simulink model "heart_model"  (Simulink 8.5)
settings: Solver=ode3  StartTime=0.0  StopTime=size(sasignal,1)  FixedStep=1  RelTol=1e-6  AbsTol=1e-6
undefined symbols (not defined in the file or in its folder): beta1, beta3, beta4, delay, gain
libraries: simulink x40, dspsrcs4 x1
(part 1 of 5)
CloseFcn:
  | rtwprivate ssgensfun ModelCloseRequest cellblocksimfast
settings Model: Creator=mereacre  LastModifiedBy=piergiuseppe  CovSFcnEnable=off
settings DataIOCC: LimitDataPoints=off  SaveOutput=off  SignalLogging=off  DSMLogging=off  SaveTime=off
settings DebuggingCC: SolverPrmCheckMsg=warning  MultiTaskDSMMsg=warning  MultiTaskCondExecSysMsg=none  FcnCallInpInsideContextMsg=EnableAllAsError
settings RTWCC: RTWCompilerOptimization=on

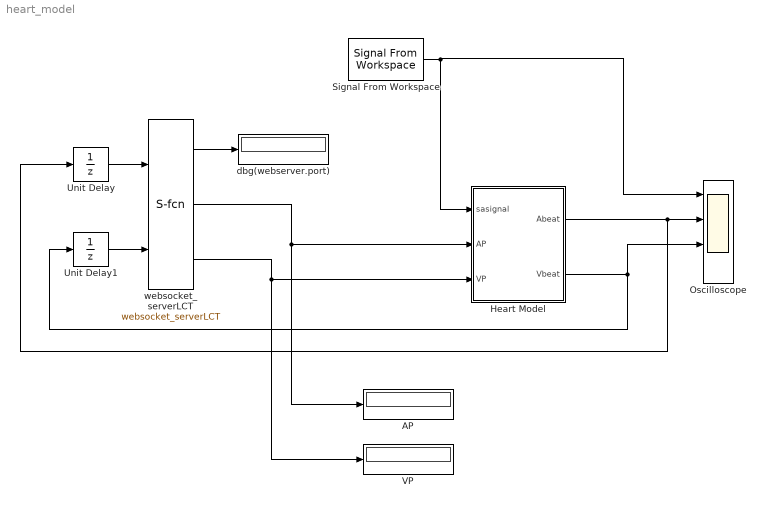
== system heart_model ==
  AP : Display
  Heart Model : Subsystem
  Oscilloscope : Scope  NumInputPorts=4
      settings: TimeRange=16384  YMin=-5~-5~-5~-5  YMax=2~5~5~5
  Signal From Workspace : dspsrcs4/Signal From Workspace  X=sasignal  Ts=1  nsamps=1  OutputAfterFinalValue=Setting to zero  ignoreOrWarnInputAndFrameLengths=off
  Unit Delay : UnitDelay  SampleTime=-1
  Unit Delay1 : UnitDelay  SampleTime=-1
  "VP " : Display
  dbg(webserver.port) : Display
  websocket_serverLCT : S-Function  FunctionName=websocket_serverLCT  mask(Legacy Function){SFunctionSpec=uint32 y1 = WebsocketServer(double u1, double u2, uint32 y2[1], uint32 y3[1]), ShowSpec=on}
      mask prompts: ShowSpec "Display function specification"
      mask help:
      | This block allows you to call the legacy functions specified by the following Legacy Code Tool definition:
      | def.SFunctionName = 'websocket_serverLCT';
      | def.OutputFcnSpec = 'uint32 y1 = WebsocketServer(double u1, double u2, uint32 y2[1], uint32 y3[1])';
      | def.TerminateFcnSpec = 'close_websocket()';
      | def.HeaderFiles = {'websocket_server.h'};
      | def.SourceFiles = {'websocket_server.c'};
      | def.HostLibFiles = {'libwebsockets.dylib'};
      mask Help: <p>This block was generated automatically by the Legacy Code Tool. For detailed help on this tool, call<a href="matlab:legacy_code('help')"> legacy_code('help')</a>.</p>
      mask Callback ShowSpec:
      | if strcmp(get_param(gcbh, 'ShowSpec'), 'on')
      |   set_param(gcbh, 'MaskDisplay', sprintf('fprintf(''%s'');', get_param(gcbh, 'SFunctionSpec')));
      | else
      |   set_param(gcbh, 'MaskDisplay', sprintf('fprintf(''%s'');', get_param(gcbh, 'FunctionName')));
      | end
      mask Display: fprintf('uint32 y1 = WebsocketServer(double u1, double u2, uint32 y2[1], uint32 y3[1])');
  wires:
  Signal From Workspace/1 -> Heart Model/1(sasignal), Oscilloscope/1
  Heart Model/2(Vbeat) -> Oscilloscope/3, Unit Delay1/1
  Heart Model/1(Abeat) -> Oscilloscope/2, Unit Delay/1
  Unit Delay1/1 -> websocket_serverLCT/2
  Unit Delay/1 -> websocket_serverLCT/1
  websocket_serverLCT/2 -> AP/1, Heart Model/2(AP)
  websocket_serverLCT/3 -> "VP "/1, Heart Model/3(VP)
  websocket_serverLCT/1 -> dbg(webserver.port)/1

== system heart_model/Heart Model ==
  sasignal : Inport
  AP : Inport  Port=2
  VP : Inport  Port=3
  ATRIUM : Subsystem
  AV (3) : Subsystem
  Action Threshold : Subsystem
  Action Threshold1 : Subsystem
  Action Threshold2 : Subsystem
  Channel ID : Constant  Value=2
  Channel ID1 : Constant  Value=2
  Constant26 : Constant  Value=0
  Constant27 : Constant  Value=gain(3)
  I_st : Constant  Value=0.7
  SA (1) : Subsystem
  VENTRICLE : Subsystem
  vin : Constant  Value=0
  Abeat : Outport
  Vbeat : Outport  Port=2
  wires:
  ATRIUM/2(scope_out) -> Action Threshold/1(v)
  Channel ID1/1 -> VENTRICLE/2(scope_in1)
  AV (3)/1(vout) -> VENTRICLE/1(vin)
  Constant27/1 -> AV (3)/4(win)
  ATRIUM/1(vout) -> AV (3)/3(vin)
  Constant26/1 -> AV (3)/2(I_st), AV (3)/1(stim)
  Channel ID/1 -> ATRIUM/2(scope_in)
  SA (1)/1(vout) -> ATRIUM/1(vin)
  vin/1 -> SA (1)/4(win), SA (1)/3(vin)
  I_st/1 -> SA (1)/2(I_st)
  sasignal/1 -> SA (1)/1(stim)
  Action Threshold/1(Aget) -> Abeat/1  "Agetsig"
  AP/1 -> ATRIUM/3(stim)
  VP/1 -> VENTRICLE/3(stim)
  VENTRICLE/1(scope_out) -> Action Threshold1/1(v), Action Threshold2/1(v)
  Action Threshold1/1(Aget) -> Vbeat/1

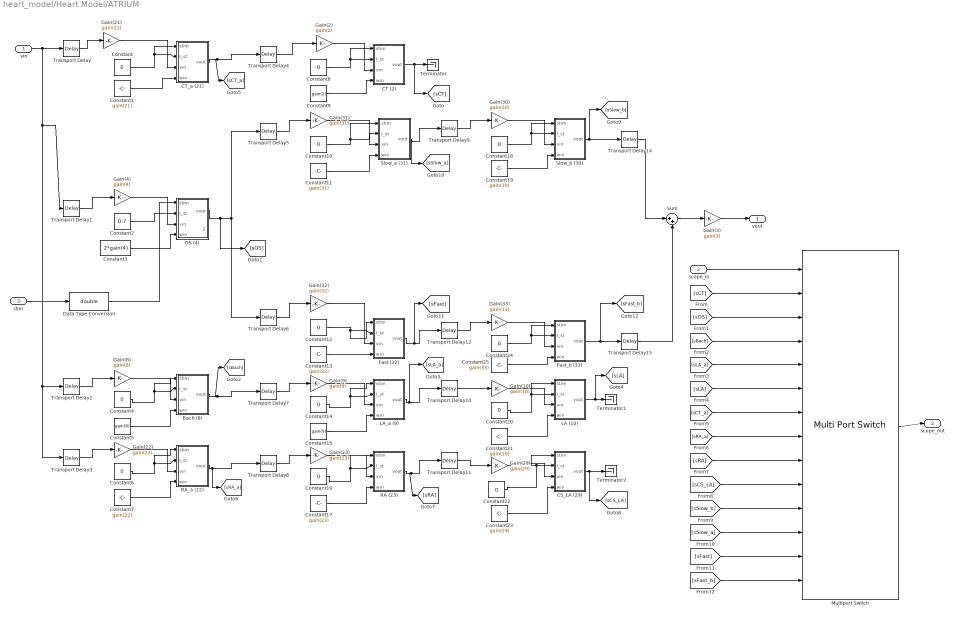
== system heart_model/Heart Model/ATRIUM ==
  vin : Inport
  scope_in : Inport  Port=2
  stim : Inport  Port=3
  Bach (8) : Subsystem
  CS_LA (29) : Subsystem
  CT (2) : Subsystem
  CT_a (21) : Subsystem
  Constant{,4,6,8,10,12,14,16,18,20,22,24} (12 alike) : Constant  Value=0
  Constant1 : Constant  Value=gain(21)
  Constant11 : Constant  Value=gain(31)
  Constant13 : Constant  Value=gain(32)
  Constant15 : Constant  Value=gain(9)
  Constant17 : Constant  Value=gain(23)
  Constant19 : Constant  Value=gain(30)
  Constant2 : Constant  Value=0.7
  Constant21 : Constant  Value=gain(10)
  Constant23 : Constant  Value=gain(29)
  Constant25 : Constant  Value=gain(33)
  Constant3 : Constant  Value=2*gain(4)
  Constant5 : Constant  Value=gain(8)
  Constant7 : Constant  Value=gain(22)
  Constant9 : Constant  Value=gain(2)
  Data Type Conversion : DataTypeConversion  OutMin=[0]  OutMax=[1]  OutDataTypeStr=double
  Fast (32) : Subsystem
  Fast_b (33) : Subsystem
  Gain(10) : Gain  Gain=gain(10)
  Gain(2) : Gain  Gain=gain(2)
  Gain(21) : Gain  Gain=gain(21)
  Gain(22) : Gain  Gain=gain(22)
  Gain(23) : Gain  Gain=gain(23)
  Gain(29) : Gain  Gain=gain(29)
  Gain(3) : Gain  Gain=gain(3)
  Gain(30) : Gain  Gain=gain(30)
  Gain(31) : Gain  Gain=gain(31)
  Gain(32) : Gain  Gain=gain(32)
  Gain(33) : Gain  Gain=gain(33)
  Gain(4) : Gain  Gain=gain(4)
  Gain(8) : Gain  Gain=gain(8)
  Gain(9) : Gain  Gain=gain(9)
  LA (10) : Subsystem
  LA_a (9) : Subsystem
  Multiport Switch : MultiPortSwitch  Inputs=13
  OS (4) : Subsystem
  RA (23) : Subsystem
  RA_a (22) : Subsystem
  Slow_a (31) : Subsystem
  Slow_b (30) : Subsystem
  Sum : Sum  Inputs=|++
  Terminator : Terminator
  Terminator1 : Terminator
  Terminator2 : Terminator
  Transport Delay : TransportDelay  DelayTime=delay(1)
  Transport Delay1 : TransportDelay  DelayTime=delay(4)
  Transport Delay10 : TransportDelay  DelayTime=delay(8)
  Transport Delay11 : TransportDelay  DelayTime=delay(30)
  Transport Delay12 : TransportDelay  DelayTime=delay(34)
  Transport Delay14 : TransportDelay  DelayTime=delay(3)
  Transport Delay15 : TransportDelay  DelayTime=delay(5)
  Transport Delay2 : TransportDelay  DelayTime=delay(6)
  Transport Delay3 : TransportDelay  DelayTime=delay(23)
  Transport Delay4 : TransportDelay  DelayTime=delay(2)
  Transport Delay5 : TransportDelay  DelayTime=delay(32)
  Transport Delay6 : TransportDelay  DelayTime=delay(33)
  Transport Delay7 : TransportDelay  DelayTime=delay(7)
  Transport Delay8 : TransportDelay  DelayTime=delay(24)
  Transport Delay9 : TransportDelay  DelayTime=delay(31)  BufferSize=3072
  vout : Outport
  scope_out : Outport  Port=2
  wires:
  Gain(4)/1 -> OS (4)/3(vin)
  Data Type Conversion/1 -> OS (4)/1(stim)
  stim/1 -> Data Type Conversion/1
  Gain(29)/1 -> CS_LA (29)/3(vin)
  Transport Delay11/1 -> Gain(29)/1
  Gain(23)/1 -> RA (23)/3(vin)
  Transport Delay8/1 -> Gain(23)/1
  Gain(22)/1 -> RA_a (22)/3(vin)
  Transport Delay3/1 -> Gain(22)/1
  Gain(10)/1 -> LA (10)/3(vin)
  Transport Delay10/1 -> Gain(10)/1
  Gain(9)/1 -> LA_a (9)/3(vin)
  Transport Delay7/1 -> Gain(9)/1
  Gain(8)/1 -> Bach (8)/3(vin)
  Transport Delay2/1 -> Gain(8)/1
  Gain(33)/1 -> Fast_b (33)/3(vin)
  Transport Delay12/1 -> Gain(33)/1
  Gain(32)/1 -> Fast (32)/3(vin)
  Transport Delay6/1 -> Gain(32)/1
  Gain(3)/1 -> vout/1
  Sum/1 -> Gain(3)/1
  Gain(30)/1 -> Slow_b (30)/3(vin)
  Transport Delay9/1 -> Gain(30)/1
  Gain(31)/1 -> Slow_a (31)/3(vin)
  Transport Delay5/1 -> Gain(31)/1
  Transport Delay1/1 -> Gain(4)/1
  Gain(2)/1 -> CT (2)/3(vin)
  Transport Delay4/1 -> Gain(2)/1
  Gain(21)/1 -> CT_a (21)/3(vin)
  Transport Delay/1 -> Gain(21)/1
  [sFast_b] -> Multiport Switch/14
  [sFast] -> Multiport Switch/13
  [sSlow_a] -> Multiport Switch/12
  [sSlow_b] -> Multiport Switch/11
  [sCS_LA] -> Multiport Switch/10
  [sRA] -> Multiport Switch/9
  [sRA_a] -> Multiport Switch/8
  [sCT_a] -> Multiport Switch/7
  [sLA] -> Multiport Switch/6
  [sLA_a] -> Multiport Switch/5
  scope_in/1 -> Multiport Switch/1
  [sBach] -> Multiport Switch/4
  [sOS] -> Multiport Switch/3
  Multiport Switch/1 -> scope_out/1
  [sCT] -> Multiport Switch/2
  Transport Delay14/1 -> Sum/1
  Transport Delay15/1 -> Sum/2
  Fast_b (33)/1(vout) -> [sFast_b], Transport Delay15/1
  Slow_b (30)/1(vout) -> [sSlow_b], Transport Delay14/1
  Fast (32)/1(vout) -> [sFast], Transport Delay12/1
  Constant25/1 -> Fast_b (33)/4(win)
  Constant24/1 -> Fast_b (33)/1(stim), Fast_b (33)/2(I_st)
  CS_LA (29)/1(vout) -> [sCS_LA], Terminator2/1
  RA (23)/1(vout) -> [sRA], Transport Delay11/1
  Constant23/1 -> CS_LA (29)/4(win)
  Constant22/1 -> CS_LA (29)/1(stim), CS_LA (29)/2(I_st)
  LA (10)/1(vout) -> [sLA], Terminator1/1
  LA_a (9)/1(vout) -> [sLA_a], Transport Delay10/1
  Constant21/1 -> LA (10)/4(win)
  Constant20/1 -> LA (10)/1(stim), LA (10)/2(I_st)
  Slow_a (31)/1(vout) -> [sSlow_a], Transport Delay9/1
  Constant19/1 -> Slow_b (30)/4(win)
  Constant18/1 -> Slow_b (30)/1(stim), Slow_b (30)/2(I_st)
  CT (2)/1(vout) -> [sCT], Terminator/1
  RA_a (22)/1(vout) -> [sRA_a], Transport Delay8/1
  Constant17/1 -> RA (23)/4(win)
  Constant16/1 -> RA (23)/1(stim), RA (23)/2(I_st)
  Bach (8)/1(vout) -> [sBach], Transport Delay7/1
  Constant15/1 -> LA_a (9)/4(win)
  Constant14/1 -> LA_a (9)/1(stim), LA_a (9)/2(I_st)
  Constant13/1 -> Fast (32)/4(win)
  Constant12/1 -> Fast (32)/1(stim), Fast (32)/2(I_st)
  OS (4)/1(vout) -> [sOS], Transport Delay6/1, Transport Delay5/1
  CT_a (21)/1(vout) -> [sCT_a], Transport Delay4/1
  Constant11/1 -> Slow_a (31)/4(win)
  Constant10/1 -> Slow_a (31)/1(stim), Slow_a (31)/2(I_st)
  Constant9/1 -> CT (2)/4(win)
  Constant8/1 -> CT (2)/1(stim), CT (2)/2(I_st)
  Constant7/1 -> RA_a (22)/4(win)
  Constant6/1 -> RA_a (22)/1(stim), RA_a (22)/2(I_st)
  Constant5/1 -> Bach (8)/4(win)
  Constant4/1 -> Bach (8)/1(stim), Bach (8)/2(I_st)
  Constant3/1 -> OS (4)/4(win)
  Constant2/1 -> OS (4)/2(I_st)
  Constant1/1 -> CT_a (21)/4(win)
  Constant/1 -> CT_a (21)/1(stim), CT_a (21)/2(I_st)
  vin/1 -> Transport Delay/1, Transport Delay1/1, Transport Delay2/1, Transport Delay3/1

== system heart_model/Heart Model/AV (3) ==
  stim : Inport
  I_st : Inport  Port=2
  vin : Inport  Port=3
  win : Inport  Port=4
  Data Type Conversion : DataTypeConversion  OutMin=[0]  OutMax=[1]  OutDataTypeStr=double  LockScale=on
  Data Type Conversion1 : DataTypeConversion  OutMin=[0]  OutMax=[1]  OutDataTypeStr=double  LockScale=on
  Data Type Conversion2 : DataTypeConversion  OutMin=[0]  OutMax=[1]  OutDataTypeStr=double  LockScale=on
  Event generator : Stateflow chart  TreatAsAtomicUnit=on
  Hybrid set : Stateflow chart  TreatAsAtomicUnit=on
  Mux : Mux  Inputs=5
  Subsystem3 : Subsystem
  vout : Outport
  wires:
  Data Type Conversion2/1 -> Mux/3
  Data Type Conversion1/1 -> Mux/2
  Event generator/3(event3) -> Data Type Conversion2/1
  Event generator/2(event2) -> Data Type Conversion1/1
  Data Type Conversion/1 -> Mux/1
  Event generator/1(event1) -> Data Type Conversion/1
  stim/1 -> Mux/5, Mux/4
  Mux/1 -> Hybrid set/Trigger
  win/1 -> Subsystem3/7(win)
  vin/1 -> Subsystem3/6(vin)
  Hybrid set/3(vno) -> Subsystem3/5(vno)
  I_st/1 -> Subsystem3/4(I_st)
  Subsystem3/1(v) -> vout/1
  Hybrid set/1(q) -> Subsystem3/1(q)
  Subsystem3/2(vnext) -> Event generator/1(v), Hybrid set/1(v)
  Hybrid set/2(vreset) -> Subsystem3/2(vreset)
  Hybrid set/4(reset) -> Subsystem3/3(reset)

== system heart_model/Heart Model/Action Threshold ==
  v : Inport
  Compare To Constant : simulink/Logic and Bit Operations/Compare To Constant  relop=>=  const=100  OutDataTypeStr=boolean
  Detect Increase : simulink/Logic and Bit Operations/Detect Increase  vinit=0.0  InputProcessing=Inherited  OutDataTypeStr=uint8
  Logical Operator : Logic  AllPortsSameDT=off  OutDataTypeStr=boolean
  ex3 : DataTypeConversion  OutMin=[0]  OutMax=[1]  OutDataTypeStr=double
  Aget : Outport
  wires:
  ex3/1 -> Aget/1
  v/1 -> Detect Increase/1, Compare To Constant/1
  Logical Operator/1 -> ex3/1
  Detect Increase/1 -> Logical Operator/2
  Compare To Constant/1 -> Logical Operator/1

== system heart_model/Heart Model/Action Threshold1 ==
  v : Inport
  Compare To Constant : simulink/Logic and Bit Operations/Compare To Constant  relop=>=  const=100  OutDataTypeStr=boolean
  Detect Increase : simulink/Logic and Bit Operations/Detect Increase  vinit=0.0  InputProcessing=Inherited  OutDataTypeStr=uint8
  Logical Operator : Logic  AllPortsSameDT=off  OutDataTypeStr=boolean
  ex3 : DataTypeConversion  OutMin=[0]  OutMax=[1]  OutDataTypeStr=double
  Aget : Outport
  wires:
  ex3/1 -> Aget/1
  v/1 -> Detect Increase/1, Compare To Constant/1
  Logical Operator/1 -> ex3/1
  Detect Increase/1 -> Logical Operator/2
  Compare To Constant/1 -> Logical Operator/1

== system heart_model/Heart Model/Action Threshold2 ==
  v : Inport
  Compare To Constant1 : simulink/Logic and Bit Operations/Compare To Constant  relop=>=  const=100  OutDataTypeStr=boolean
  Compare To Constant2 : simulink/Logic and Bit Operations/Compare To Constant  relop=<=  const=102  OutDataTypeStr=boolean
  Detect Increase1 : simulink/Logic and Bit Operations/Detect Increase  vinit=0.0  InputProcessing=Inherited  OutDataTypeStr=uint8
  Logical Operator1 : Logic  AllPortsSameDT=off  OutDataTypeStr=boolean
  Logical Operator2 : Logic  Operator=OR  AllPortsSameDT=off  OutDataTypeStr=boolean
  ex3 : DataTypeConversion  OutMin=[0]  OutMax=[1]  OutDataTypeStr=double  RndMeth=Convergent  LockScale=on
  Vget : Outport
  wires:
  ex3/1 -> Vget/1
  Logical Operator1/1 -> Logical Operator2/1
  Compare To Constant1/1 -> Logical Operator1/1
  Detect Increase1/1 -> Logical Operator1/2
  v/1 -> Compare To Constant1/1, Detect Increase1/1, Compare To Constant2/1
  Compare To Constant2/1 -> Logical Operator2/2
  Logical Operator2/1 -> ex3/1

== system heart_model/Heart Model/SA (1) ==
  stim : Inport
  I_st : Inport  Port=2
  vin : Inport  Port=3
  win : Inport  Port=4
  Data Type Conversion : DataTypeConversion  OutMin=[0]  OutMax=[1]  OutDataTypeStr=double  LockScale=on
  Data Type Conversion1 : DataTypeConversion  OutMin=[0]  OutMax=[1]  OutDataTypeStr=double  LockScale=on
  Data Type Conversion2 : DataTypeConversion  OutMin=[0]  OutMax=[1]  OutDataTypeStr=double  LockScale=on
  Event generator : Stateflow chart  TreatAsAtomicUnit=on
  Hybrid set : Stateflow chart  TreatAsAtomicUnit=on
  Mux : Mux  Inputs=5
  Subsystem3 : Subsystem
  vout : Outport
  wires:
  Data Type Conversion2/1 -> Mux/3
  Data Type Conversion1/1 -> Mux/2
  Event generator/3(event3) -> Data Type Conversion2/1
  Event generator/2(event2) -> Data Type Conversion1/1
  Data Type Conversion/1 -> Mux/1
  Event generator/1(event1) -> Data Type Conversion/1
  stim/1 -> Mux/5, Mux/4
  Mux/1 -> Hybrid set/Trigger
  win/1 -> Subsystem3/7(win)
  vin/1 -> Subsystem3/6(vin)
  Hybrid set/3(vno) -> Subsystem3/5(vno)
  I_st/1 -> Subsystem3/4(I_st)
  Subsystem3/1(v) -> vout/1
  Hybrid set/1(q) -> Subsystem3/1(q)
  Subsystem3/2(vnext) -> Event generator/1(v), Hybrid set/1(v)
  Hybrid set/2(vreset) -> Subsystem3/2(vreset)
  Hybrid set/4(reset) -> Subsystem3/3(reset)

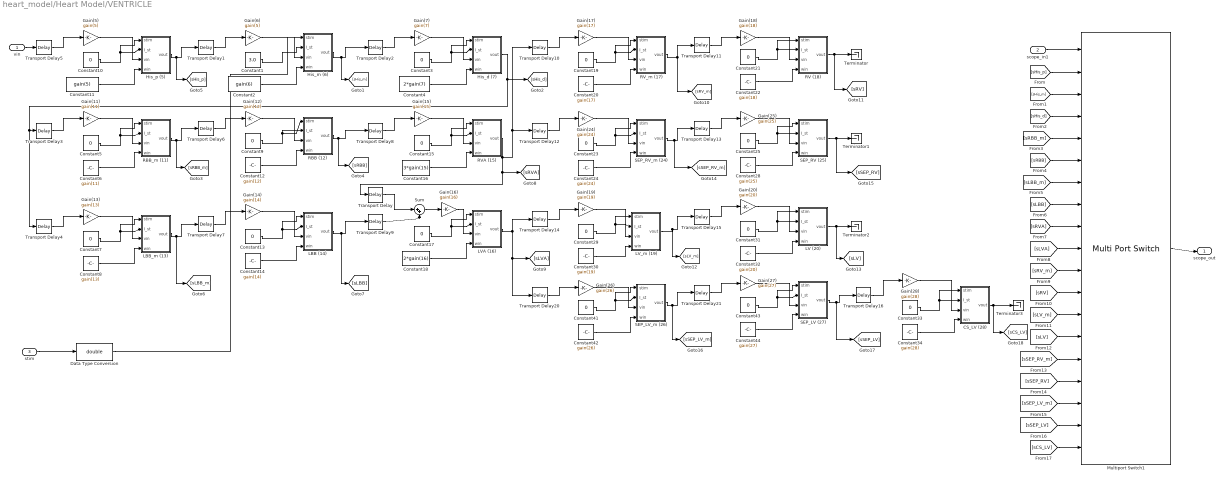
== system heart_model/Heart Model/VENTRICLE ==
  vin : Inport
  scope_in1 : Inport  Port=2
  stim : Inport  Port=3
  CS_LV (28) : Subsystem
  Constant1 : Constant  Value=3.0
  Constant{3,5,7,9..10,13,15,17,19,21,23,25,29,31,33,41,43} (17 alike) : Constant  Value=0
  Constant11 : Constant  Value=gain(5)
  Constant12 : Constant  Value=gain(12)
  Constant14 : Constant  Value=gain(14)
  Constant16 : Constant  Value=3*gain(15)
  Constant18 : Constant  Value=2*gain(16)
  Constant2 : Constant  Value=gain(6)
  Constant20 : Constant  Value=gain(17)
  Constant22 : Constant  Value=gain(18)
  Constant24 : Constant  Value=gain(24)
  Constant28 : Constant  Value=gain(25)
  Constant30 : Constant  Value=gain(19)
  Constant32 : Constant  Value=gain(20)
  Constant34 : Constant  Value=gain(28)
  Constant4 : Constant  Value=2*gain(7)
  Constant42 : Constant  Value=gain(26)
  Constant44 : Constant  Value=gain(27)
  Constant6 : Constant  Value=gain(11)
  Constant8 : Constant  Value=gain(13)
  Data Type Conversion : DataTypeConversion  OutMin=[0]  OutMax=[1]  OutDataTypeStr=double
  Gain(11) : Gain  Gain=gain(11)
  Gain(12) : Gain  Gain=gain(12)
  Gain(13) : Gain  Gain=gain(13)
  Gain(14) : Gain  Gain=gain(14)
  Gain(15) : Gain  Gain=gain(15)
  Gain(16) : Gain  Gain=gain(16)
  Gain(17) : Gain  Gain=gain(17)
  Gain(18) : Gain  Gain=gain(18)
  Gain(19) : Gain  Gain=gain(19)
  Gain(20) : Gain  Gain=gain(20)
  Gain(24) : Gain  Gain=gain(24)
  Gain(25) : Gain  Gain=gain(25)
  Gain(26) : Gain  Gain=gain(26)
  Gain(27) : Gain  Gain=gain(27)
  Gain(28) : Gain  Gain=gain(28)
  Gain(5) : Gain  Gain=gain(5)
  Gain(6) : Gain  Gain=gain(5)
  Gain(7) : Gain  Gain=gain(7)
  His_d (7) : Subsystem
  His_m (6) : Subsystem
  His_p (5) : Subsystem
  LBB (14) : Subsystem
  LBB_m (13) : Subsystem
  LV (20) : Subsystem
  LVA (16) : Subsystem
  LV_m (19) : Subsystem
  Multiport Switch1 : MultiPortSwitch  Inputs=18
  RBB (12) : Subsystem
  RBB_m (11) : Subsystem
  RV (18) : Subsystem
  RVA (15) : Subsystem
  RV_m (17) : Subsystem
  SEP_LV (27) : Subsystem
  SEP_LV_m (26) : Subsystem
  SEP_RV (25) : Subsystem
  SEP_RV_m (24) : Subsystem
  Sum : Sum  Inputs=|++
  Terminator{,1..3} (4 alike) : Terminator
  Transport Delay : TransportDelay  DelayTime=delay(18)
  Transport Delay1 : TransportDelay  DelayTime=delay(10)
  Transport Delay10 : TransportDelay  DelayTime=delay(19)
  Transport Delay11 : TransportDelay  DelayTime=delay(21)
  Transport Delay12 : TransportDelay  DelayTime=delay(26)
  Transport Delay13 : TransportDelay  DelayTime=delay(25)
  Transport Delay14 : TransportDelay  DelayTime=delay(20)
  Transport Delay15 : TransportDelay  DelayTime=delay(22)
  Transport Delay16 : TransportDelay  DelayTime=delay(29)
  Transport Delay2 : TransportDelay  DelayTime=delay(11)
  Transport Delay20 : TransportDelay  DelayTime=delay(28)
  Transport Delay21 : TransportDelay  DelayTime=delay(27)
  Transport Delay3 : TransportDelay  DelayTime=delay(12)
  Transport Delay4 : TransportDelay  DelayTime=delay(13)
  Transport Delay5 : TransportDelay  DelayTime=delay(9)
  Transport Delay6 : TransportDelay  DelayTime=delay(14)
  Transport Delay7 : TransportDelay  DelayTime=delay(15)
  Transport Delay8 : TransportDelay  DelayTime=delay(16)
  Transport Delay9 : TransportDelay  DelayTime=delay(17)
  scope_out : Outport
  wires:
  Data Type Conversion/1 -> His_m (6)/1(stim)
  stim/1 -> Data Type Conversion/1
  Gain(28)/1 -> CS_LV (28)/3(vin)
  Transport Delay16/1 -> Gain(28)/1
  Gain(27)/1 -> SEP_LV (27)/3(vin)
  Transport Delay21/1 -> Gain(27)/1
  Gain(20)/1 -> LV (20)/3(vin)
  Transport Delay15/1 -> Gain(20)/1
  Gain(26)/1 -> SEP_LV_m (26)/3(vin)
  Transport Delay20/1 -> Gain(26)/1
  Gain(19)/1 -> LV_m (19)/3(vin)
  Transport Delay14/1 -> Gain(19)/1
  Gain(16)/1 -> LVA (16)/3(vin)
  Sum/1 -> Gain(16)/1
  Gain(14)/1 -> LBB (14)/3(vin)
  Transport Delay7/1 -> Gain(14)/1
  Gain(13)/1 -> LBB_m (13)/3(vin)
  Transport Delay4/1 -> Gain(13)/1
  Gain(25)/1 -> SEP_RV (25)/3(vin)
  Transport Delay13/1 -> Gain(25)/1
  Gain(24)/1 -> SEP_RV_m (24)/3(vin)
  Transport Delay12/1 -> Gain(24)/1
  Gain(15)/1 -> RVA (15)/3(vin)
  Transport Delay8/1 -> Gain(15)/1
  Gain(12)/1 -> RBB (12)/3(vin)
  Transport Delay6/1 -> Gain(12)/1
  Gain(11)/1 -> RBB_m (11)/3(vin)
  Transport Delay3/1 -> Gain(11)/1
  Gain(18)/1 -> RV (18)/3(vin)
  Transport Delay11/1 -> Gain(18)/1
  Gain(17)/1 -> RV_m (17)/3(vin)
  Transport Delay10/1 -> Gain(17)/1
  Gain(7)/1 -> His_d (7)/3(vin)
  Transport Delay2/1 -> Gain(7)/1
  Gain(6)/1 -> His_m (6)/3(vin)
  Transport Delay1/1 -> Gain(6)/1
  Gain(5)/1 -> His_p (5)/3(vin)
  Transport Delay5/1 -> Gain(5)/1
  [sCS_LV] -> Multiport Switch1/19
  [sSEP_LV] -> Multiport Switch1/18
  [sSEP_LV_m] -> Multiport Switch1/17
  [sSEP_RV] -> Multiport Switch1/16
  [sSEP_RV_m] -> Multiport Switch1/15
  [sLV] -> Multiport Switch1/14
  [sLV_m] -> Multiport Switch1/13
  [sRV] -> Multiport Switch1/12
  [sRV_m] -> Multiport Switch1/11
  [sLVA] -> Multiport Switch1/10
  [sRVA] -> Multiport Switch1/9
  [sLBB] -> Multiport Switch1/8
  [sLBB_m] -> Multiport Switch1/7
  [sRBB] -> Multiport Switch1/6
  [sRBB_m] -> Multiport Switch1/5
  scope_in1/1 -> Multiport Switch1/1
  [sHis_d] -> Multiport Switch1/4
  [sHis_m] -> Multiport Switch1/3
  Multiport Switch1/1 -> scope_out/1
  [sHis_p] -> Multiport Switch1/2
  vin/1 -> Transport Delay5/1
  CS_LV (28)/1(vout) -> [sCS_LV], Terminator3/1
  SEP_LV (27)/1(vout) -> [sSEP_LV], Transport Delay16/1
  Constant34/1 -> CS_LV (28)/4(win)
  Constant33/1 -> CS_LV (28)/2(I_st), CS_LV (28)/1(stim)
  SEP_LV_m (26)/1(vout) -> [sSEP_LV_m], Transport Delay21/1
  Constant44/1 -> SEP_LV (27)/4(win)
  Constant43/1 -> SEP_LV (27)/2(I_st), SEP_LV (27)/1(stim)
  Constant42/1 -> SEP_LV_m (26)/4(win)
  Constant41/1 -> SEP_LV_m (26)/2(I_st), SEP_LV_m (26)/1(stim)
  LV (20)/1(vout) -> [sLV], Terminator2/1
  LV_m (19)/1(vout) -> [sLV_m], Transport Delay15/1
  Constant32/1 -> LV (20)/4(win)
  Constant31/1 -> LV (20)/2(I_st), LV (20)/1(stim)
  LVA (16)/1(vout) -> [sLVA], Transport Delay20/1, Transport Delay14/1
  Constant30/1 -> LV_m (19)/4(win)
  Constant29/1 -> LV_m (19)/2(I_st), LV_m (19)/1(stim)
  SEP_RV (25)/1(vout) -> [sSEP_RV], Terminator1/1
  SEP_RV_m (24)/1(vout) -> [sSEP_RV_m], Transport Delay13/1
  Constant28/1 -> SEP_RV (25)/4(win)
  Constant25/1 -> SEP_RV (25)/2(I_st), SEP_RV (25)/1(stim)
  Constant24/1 -> SEP_RV_m (24)/4(win)
  Constant23/1 -> SEP_RV_m (24)/2(I_st), SEP_RV_m (24)/1(stim)
  RV (18)/1(vout) -> [sRV], Terminator/1
  RV_m (17)/1(vout) -> [sRV_m], Transport Delay11/1
  Constant22/1 -> RV (18)/4(win)
  Constant21/1 -> RV (18)/2(I_st), RV (18)/1(stim)
  Constant20/1 -> RV_m (17)/4(win)
  Constant19/1 -> RV_m (17)/2(I_st), RV_m (17)/1(stim)
  RVA (15)/1(vout) -> [sRVA], Transport Delay/1, Transport Delay10/1, Transport Delay12/1
  Transport Delay9/1 -> Sum/2
  Transport Delay/1 -> Sum/1
  LBB (14)/1(vout) -> [sLBB], Transport Delay9/1
  Constant18/1 -> LVA (16)/4(win)
  Constant17/1 -> LVA (16)/2(I_st), LVA (16)/1(stim)
  RBB (12)/1(vout) -> [sRBB], Transport Delay8/1
  Constant16/1 -> RVA (15)/4(win)
  Constant15/1 -> RVA (15)/2(I_st), RVA (15)/1(stim)
  LBB_m (13)/1(vout) -> [sLBB_m], Transport Delay7/1
  Constant14/1 -> LBB (14)/4(win)
  Constant13/1 -> LBB (14)/2(I_st), LBB (14)/1(stim)
  RBB_m (11)/1(vout) -> [sRBB_m], Transport Delay6/1
  Constant12/1 -> RBB (12)/4(win)
  Constant9/1 -> RBB (12)/2(I_st), RBB (12)/1(stim)
  Constant8/1 -> LBB_m (13)/4(win)
  Constant7/1 -> LBB_m (13)/2(I_st), LBB_m (13)/1(stim)
  His_d (7)/1(vout) -> [sHis_d], Transport Delay4/1, Transport Delay3/1
  Constant6/1 -> RBB_m (11)/4(win)
  Constant5/1 -> RBB_m (11)/2(I_st), RBB_m (11)/1(stim)
  His_m (6)/1(vout) -> [sHis_m], Transport Delay2/1
  Constant4/1 -> His_d (7)/4(win)
  Constant3/1 -> His_d (7)/2(I_st), His_d (7)/1(stim)
  His_p (5)/1(vout) -> Transport Delay1/1, [sHis_p]
  Constant2/1 -> His_m (6)/4(win)
  Constant1/1 -> His_m (6)/2(I_st)
  Constant11/1 -> His_p (5)/4(win)
  Constant10/1 -> His_p (5)/2(I_st), His_p (5)/1(stim)

== system heart_model/Heart Model/ATRIUM/Bach (8) ==
  stim : Inport
  I_st : Inport  Port=2
  vin : Inport  Port=3
  win : Inport  Port=4
  Data Type Conversion : DataTypeConversion  OutMin=[0]  OutMax=[1]  OutDataTypeStr=double  LockScale=on
  Data Type Conversion1 : DataTypeConversion  OutMin=[0]  OutMax=[1]  OutDataTypeStr=double  LockScale=on
  Data Type Conversion2 : DataTypeConversion  OutMin=[0]  OutMax=[1]  OutDataTypeStr=double  LockScale=on
  Event generator : Stateflow chart  TreatAsAtomicUnit=on
  Hybrid set : Stateflow chart  TreatAsAtomicUnit=on
  Mux : Mux  Inputs=5
  Subsystem3 : Subsystem
  vout : Outport
  wires:
  Data Type Conversion2/1 -> Mux/3
  Data Type Conversion1/1 -> Mux/2
  Event generator/3(event3) -> Data Type Conversion2/1
  Event generator/2(event2) -> Data Type Conversion1/1
  Data Type Conversion/1 -> Mux/1
  Event generator/1(event1) -> Data Type Conversion/1
  stim/1 -> Mux/5, Mux/4
  Mux/1 -> Hybrid set/Trigger
  win/1 -> Subsystem3/7(win)
  vin/1 -> Subsystem3/6(vin)
  Hybrid set/3(vno) -> Subsystem3/5(vno)
  I_st/1 -> Subsystem3/4(I_st)
  Subsystem3/1(v) -> vout/1
  Hybrid set/1(q) -> Subsystem3/1(q)
  Subsystem3/2(vnext) -> Event generator/1(v), Hybrid set/1(v)
  Hybrid set/2(vreset) -> Subsystem3/2(vreset)
  Hybrid set/4(reset) -> Subsystem3/3(reset)

== system heart_model/Heart Model/ATRIUM/CS_LA (29) ==
  stim : Inport
  I_st : Inport  Port=2
  vin : Inport  Port=3
  win : Inport  Port=4
  Data Type Conversion : DataTypeConversion  OutMin=[0]  OutMax=[1]  OutDataTypeStr=double  LockScale=on
  Data Type Conversion1 : DataTypeConversion  OutMin=[0]  OutMax=[1]  OutDataTypeStr=double  LockScale=on
  Data Type Conversion2 : DataTypeConversion  OutMin=[0]  OutMax=[1]  OutDataTypeStr=double  LockScale=on
  Event generator : Stateflow chart  TreatAsAtomicUnit=on
  Hybrid set : Stateflow chart  TreatAsAtomicUnit=on
  Mux : Mux  Inputs=5
  Subsystem3 : Subsystem
  vout : Outport
  wires:
  Data Type Conversion2/1 -> Mux/3
  Data Type Conversion1/1 -> Mux/2
  Event generator/3(event3) -> Data Type Conversion2/1
  Event generator/2(event2) -> Data Type Conversion1/1
  Data Type Conversion/1 -> Mux/1
  Event generator/1(event1) -> Data Type Conversion/1
  stim/1 -> Mux/5, Mux/4
  Mux/1 -> Hybrid set/Trigger
  win/1 -> Subsystem3/7(win)
  vin/1 -> Subsystem3/6(vin)
  Hybrid set/3(vno) -> Subsystem3/5(vno)
  I_st/1 -> Subsystem3/4(I_st)
  Subsystem3/1(v) -> vout/1
  Hybrid set/1(q) -> Subsystem3/1(q)
  Subsystem3/2(vnext) -> Event generator/1(v), Hybrid set/1(v)
  Hybrid set/2(vreset) -> Subsystem3/2(vreset)
  Hybrid set/4(reset) -> Subsystem3/3(reset)

== system heart_model/Heart Model/ATRIUM/CT (2) ==
  stim : Inport
  I_st : Inport  Port=2
  vin : Inport  Port=3
  win : Inport  Port=4
  Data Type Conversion : DataTypeConversion  OutMin=[0]  OutMax=[1]  OutDataTypeStr=double  LockScale=on
  Data Type Conversion1 : DataTypeConversion  OutMin=[0]  OutMax=[1]  OutDataTypeStr=double  LockScale=on
  Data Type Conversion2 : DataTypeConversion  OutMin=[0]  OutMax=[1]  OutDataTypeStr=double  LockScale=on
  Event generator : Stateflow chart  TreatAsAtomicUnit=on
  Hybrid set : Stateflow chart  TreatAsAtomicUnit=on
  Mux : Mux  Inputs=5
  Subsystem3 : Subsystem
  vout : Outport
  wires:
  Data Type Conversion2/1 -> Mux/3
  Data Type Conversion1/1 -> Mux/2
  Event generator/3(event3) -> Data Type Conversion2/1
  Event generator/2(event2) -> Data Type Conversion1/1
  Data Type Conversion/1 -> Mux/1
  Event generator/1(event1) -> Data Type Conversion/1
  stim/1 -> Mux/5, Mux/4
  Mux/1 -> Hybrid set/Trigger
  win/1 -> Subsystem3/7(win)
  vin/1 -> Subsystem3/6(vin)
  Hybrid set/3(vno) -> Subsystem3/5(vno)
  I_st/1 -> Subsystem3/4(I_st)
  Subsystem3/1(v) -> vout/1
  Hybrid set/1(q) -> Subsystem3/1(q)
  Subsystem3/2(vnext) -> Event generator/1(v), Hybrid set/1(v)
  Hybrid set/2(vreset) -> Subsystem3/2(vreset)
  Hybrid set/4(reset) -> Subsystem3/3(reset)

== system heart_model/Heart Model/ATRIUM/CT_a (21) ==
  stim : Inport
  I_st : Inport  Port=2
  vin : Inport  Port=3
  win : Inport  Port=4
  Data Type Conversion : DataTypeConversion  OutMin=[0]  OutMax=[1]  OutDataTypeStr=double  LockScale=on
  Data Type Conversion1 : DataTypeConversion  OutMin=[0]  OutMax=[1]  OutDataTypeStr=double  LockScale=on
  Data Type Conversion2 : DataTypeConversion  OutMin=[0]  OutMax=[1]  OutDataTypeStr=double  LockScale=on
  Event generator : Stateflow chart  TreatAsAtomicUnit=on
  Hybrid set : Stateflow chart  TreatAsAtomicUnit=on
  Mux : Mux  Inputs=5
  Subsystem3 : Subsystem
  vout : Outport
  wires:
  Data Type Conversion2/1 -> Mux/3
  Data Type Conversion1/1 -> Mux/2
  Event generator/3(event3) -> Data Type Conversion2/1
  Event generator/2(event2) -> Data Type Conversion1/1
  Data Type Conversion/1 -> Mux/1
  Event generator/1(event1) -> Data Type Conversion/1
  stim/1 -> Mux/5, Mux/4
  Mux/1 -> Hybrid set/Trigger
  win/1 -> Subsystem3/7(win)
  vin/1 -> Subsystem3/6(vin)
  Hybrid set/3(vno) -> Subsystem3/5(vno)
  I_st/1 -> Subsystem3/4(I_st)
  Subsystem3/1(v) -> vout/1
  Hybrid set/1(q) -> Subsystem3/1(q)
  Subsystem3/2(vnext) -> Event generator/1(v), Hybrid set/1(v)
  Hybrid set/2(vreset) -> Subsystem3/2(vreset)
  Hybrid set/4(reset) -> Subsystem3/3(reset)

== system heart_model/Heart Model/ATRIUM/Fast (32) ==
  stim : Inport
  I_st : Inport  Port=2
  vin : Inport  Port=3
  win : Inport  Port=4
  Data Type Conversion : DataTypeConversion  OutMin=[0]  OutMax=[1]  OutDataTypeStr=double  LockScale=on
  Data Type Conversion1 : DataTypeConversion  OutMin=[0]  OutMax=[1]  OutDataTypeStr=double  LockScale=on
  Data Type Conversion2 : DataTypeConversion  OutMin=[0]  OutMax=[1]  OutDataTypeStr=double  LockScale=on
  Event generator : Stateflow chart  TreatAsAtomicUnit=on
  Hybrid set : Stateflow chart  TreatAsAtomicUnit=on
  Mux : Mux  Inputs=5
  Subsystem3 : Subsystem
  vout : Outport
  wires:
  Data Type Conversion2/1 -> Mux/3
  Data Type Conversion1/1 -> Mux/2
  Event generator/3(event3) -> Data Type Conversion2/1
  Event generator/2(event2) -> Data Type Conversion1/1
  Data Type Conversion/1 -> Mux/1
  Event generator/1(event1) -> Data Type Conversion/1
  stim/1 -> Mux/5, Mux/4
  Mux/1 -> Hybrid set/Trigger
  win/1 -> Subsystem3/7(win)
  vin/1 -> Subsystem3/6(vin)
  Hybrid set/3(vno) -> Subsystem3/5(vno)
  I_st/1 -> Subsystem3/4(I_st)
  Subsystem3/1(v) -> vout/1
  Hybrid set/1(q) -> Subsystem3/1(q)
  Subsystem3/2(vnext) -> Event generator/1(v), Hybrid set/1(v)
  Hybrid set/2(vreset) -> Subsystem3/2(vreset)
  Hybrid set/4(reset) -> Subsystem3/3(reset)

== system heart_model/Heart Model/ATRIUM/Fast_b (33) ==
  stim : Inport
  I_st : Inport  Port=2
  vin : Inport  Port=3
  win : Inport  Port=4
  Data Type Conversion : DataTypeConversion  OutMin=[0]  OutMax=[1]  OutDataTypeStr=double  LockScale=on
  Data Type Conversion1 : DataTypeConversion  OutMin=[0]  OutMax=[1]  OutDataTypeStr=double  LockScale=on
  Data Type Conversion2 : DataTypeConversion  OutMin=[0]  OutMax=[1]  OutDataTypeStr=double  LockScale=on
  Event generator : Stateflow chart  TreatAsAtomicUnit=on
  Hybrid set : Stateflow chart  TreatAsAtomicUnit=on
  Mux : Mux  Inputs=5
  Subsystem3 : Subsystem
  vout : Outport
  wires:
  Data Type Conversion2/1 -> Mux/3
  Data Type Conversion1/1 -> Mux/2
  Event generator/3(event3) -> Data Type Conversion2/1
  Event generator/2(event2) -> Data Type Conversion1/1
  Data Type Conversion/1 -> Mux/1
  Event generator/1(event1) -> Data Type Conversion/1
  stim/1 -> Mux/5, Mux/4
  Mux/1 -> Hybrid set/Trigger
  win/1 -> Subsystem3/7(win)
  vin/1 -> Subsystem3/6(vin)
  Hybrid set/3(vno) -> Subsystem3/5(vno)
  I_st/1 -> Subsystem3/4(I_st)
  Subsystem3/1(v) -> vout/1
  Hybrid set/1(q) -> Subsystem3/1(q)
  Subsystem3/2(vnext) -> Event generator/1(v), Hybrid set/1(v)
  Hybrid set/2(vreset) -> Subsystem3/2(vreset)
  Hybrid set/4(reset) -> Subsystem3/3(reset)

== system heart_model/Heart Model/ATRIUM/LA (10) ==
  stim : Inport
  I_st : Inport  Port=2
  vin : Inport  Port=3
  win : Inport  Port=4
  Data Type Conversion : DataTypeConversion  OutMin=[0]  OutMax=[1]  OutDataTypeStr=double  LockScale=on
  Data Type Conversion1 : DataTypeConversion  OutMin=[0]  OutMax=[1]  OutDataTypeStr=double  LockScale=on
  Data Type Conversion2 : DataTypeConversion  OutMin=[0]  OutMax=[1]  OutDataTypeStr=double  LockScale=on
  Event generator : Stateflow chart  TreatAsAtomicUnit=on
  Hybrid set : Stateflow chart  TreatAsAtomicUnit=on
  Mux : Mux  Inputs=5
  Subsystem3 : Subsystem
  vout : Outport
  wires:
  Data Type Conversion2/1 -> Mux/3
  Data Type Conversion1/1 -> Mux/2
  Event generator/3(event3) -> Data Type Conversion2/1
  Event generator/2(event2) -> Data Type Conversion1/1
  Data Type Conversion/1 -> Mux/1
  Event generator/1(event1) -> Data Type Conversion/1
  stim/1 -> Mux/5, Mux/4
  Mux/1 -> Hybrid set/Trigger
  win/1 -> Subsystem3/7(win)
  vin/1 -> Subsystem3/6(vin)
  Hybrid set/3(vno) -> Subsystem3/5(vno)
  I_st/1 -> Subsystem3/4(I_st)
  Subsystem3/1(v) -> vout/1
  Hybrid set/1(q) -> Subsystem3/1(q)
  Subsystem3/2(vnext) -> Event generator/1(v), Hybrid set/1(v)
  Hybrid set/2(vreset) -> Subsystem3/2(vreset)
  Hybrid set/4(reset) -> Subsystem3/3(reset)

== system heart_model/Heart Model/ATRIUM/LA_a (9) ==
  stim : Inport
  I_st : Inport  Port=2
  vin : Inport  Port=3
  win : Inport  Port=4
  Data Type Conversion : DataTypeConversion  OutMin=[0]  OutMax=[1]  OutDataTypeStr=double  LockScale=on
  Data Type Conversion1 : DataTypeConversion  OutMin=[0]  OutMax=[1]  OutDataTypeStr=double  LockScale=on
  Data Type Conversion2 : DataTypeConversion  OutMin=[0]  OutMax=[1]  OutDataTypeStr=double  LockScale=on
  Event generator : Stateflow chart  TreatAsAtomicUnit=on
  Hybrid set : Stateflow chart  TreatAsAtomicUnit=on
  Mux : Mux  Inputs=5
  Subsystem3 : Subsystem
  vout : Outport
  wires:
  Data Type Conversion2/1 -> Mux/3
  Data Type Conversion1/1 -> Mux/2
  Event generator/3(event3) -> Data Type Conversion2/1
  Event generator/2(event2) -> Data Type Conversion1/1
  Data Type Conversion/1 -> Mux/1
  Event generator/1(event1) -> Data Type Conversion/1
  stim/1 -> Mux/5, Mux/4
  Mux/1 -> Hybrid set/Trigger
  win/1 -> Subsystem3/7(win)
  vin/1 -> Subsystem3/6(vin)
  Hybrid set/3(vno) -> Subsystem3/5(vno)
  I_st/1 -> Subsystem3/4(I_st)
  Subsystem3/1(v) -> vout/1
  Hybrid set/1(q) -> Subsystem3/1(q)
  Subsystem3/2(vnext) -> Event generator/1(v), Hybrid set/1(v)
  Hybrid set/2(vreset) -> Subsystem3/2(vreset)
  Hybrid set/4(reset) -> Subsystem3/3(reset)

== system heart_model/Heart Model/ATRIUM/OS (4) ==
  stim : Inport
  I_st : Inport  Port=2
  vin : Inport  Port=3
  win : Inport  Port=4
  Data Type Conversion : DataTypeConversion  OutMin=[0]  OutMax=[1]  OutDataTypeStr=double  LockScale=on
  Data Type Conversion1 : DataTypeConversion  OutMin=[0]  OutMax=[1]  OutDataTypeStr=double  LockScale=on
  Data Type Conversion2 : DataTypeConversion  OutMin=[0]  OutMax=[1]  OutDataTypeStr=double  LockScale=on
  Event generator : Stateflow chart  TreatAsAtomicUnit=on
  Hybrid set : Stateflow chart  TreatAsAtomicUnit=on
  Mux : Mux  Inputs=5
  Subsystem3 : Subsystem
  vout : Outport
  vnext : Outport  Port=2
  wires:
  Data Type Conversion2/1 -> Mux/3
  Data Type Conversion1/1 -> Mux/2
  Event generator/3(event3) -> Data Type Conversion2/1
  Event generator/2(event2) -> Data Type Conversion1/1
  Data Type Conversion/1 -> Mux/1
  Event generator/1(event1) -> Data Type Conversion/1
  stim/1 -> Mux/5, Mux/4
  Mux/1 -> Hybrid set/Trigger
  win/1 -> Subsystem3/7(win)
  vin/1 -> Subsystem3/6(vin)
  Hybrid set/3(vno) -> Subsystem3/5(vno)
  I_st/1 -> Subsystem3/4(I_st)
  Subsystem3/1(v) -> vout/1
  Hybrid set/1(q) -> Subsystem3/1(q)
  Subsystem3/2(vnext) -> vnext/1, Event generator/1(v), Hybrid set/1(v)
  Hybrid set/2(vreset) -> Subsystem3/2(vreset)
  Hybrid set/4(reset) -> Subsystem3/3(reset)

== system heart_model/Heart Model/ATRIUM/RA (23) ==
  stim : Inport
  I_st : Inport  Port=2
  vin : Inport  Port=3
  win : Inport  Port=4
  Data Type Conversion : DataTypeConversion  OutMin=[0]  OutMax=[1]  OutDataTypeStr=double  LockScale=on
  Data Type Conversion1 : DataTypeConversion  OutMin=[0]  OutMax=[1]  OutDataTypeStr=double  LockScale=on
  Data Type Conversion2 : DataTypeConversion  OutMin=[0]  OutMax=[1]  OutDataTypeStr=double  LockScale=on
  Event generator : Stateflow chart  TreatAsAtomicUnit=on
  Hybrid set : Stateflow chart  TreatAsAtomicUnit=on
  Mux : Mux  Inputs=5
  Subsystem3 : Subsystem
  vout : Outport
  wires:
  Data Type Conversion2/1 -> Mux/3
  Data Type Conversion1/1 -> Mux/2
  Event generator/3(event3) -> Data Type Conversion2/1
  Event generator/2(event2) -> Data Type Conversion1/1
  Data Type Conversion/1 -> Mux/1
  Event generator/1(event1) -> Data Type Conversion/1
  stim/1 -> Mux/5, Mux/4
  Mux/1 -> Hybrid set/Trigger
  win/1 -> Subsystem3/7(win)
  vin/1 -> Subsystem3/6(vin)
  Hybrid set/3(vno) -> Subsystem3/5(vno)
  I_st/1 -> Subsystem3/4(I_st)
  Subsystem3/1(v) -> vout/1
  Hybrid set/1(q) -> Subsystem3/1(q)
  Subsystem3/2(vnext) -> Event generator/1(v), Hybrid set/1(v)
  Hybrid set/2(vreset) -> Subsystem3/2(vreset)
  Hybrid set/4(reset) -> Subsystem3/3(reset)

== system heart_model/Heart Model/ATRIUM/RA_a (22) ==
  stim : Inport
  I_st : Inport  Port=2
  vin : Inport  Port=3
  win : Inport  Port=4
  Data Type Conversion : DataTypeConversion  OutMin=[0]  OutMax=[1]  OutDataTypeStr=double  LockScale=on
  Data Type Conversion1 : DataTypeConversion  OutMin=[0]  OutMax=[1]  OutDataTypeStr=double  LockScale=on
  Data Type Conversion2 : DataTypeConversion  OutMin=[0]  OutMax=[1]  OutDataTypeStr=double  LockScale=on
  Event generator : Stateflow chart  TreatAsAtomicUnit=on
  Hybrid set : Stateflow chart  TreatAsAtomicUnit=on
  Mux : Mux  Inputs=5
  Subsystem3 : Subsystem
  vout : Outport
  wires:
  Data Type Conversion2/1 -> Mux/3
  Data Type Conversion1/1 -> Mux/2
  Event generator/3(event3) -> Data Type Conversion2/1
  Event generator/2(event2) -> Data Type Conversion1/1
  Data Type Conversion/1 -> Mux/1
  Event generator/1(event1) -> Data Type Conversion/1
  stim/1 -> Mux/5, Mux/4
  Mux/1 -> Hybrid set/Trigger
  win/1 -> Subsystem3/7(win)
  vin/1 -> Subsystem3/6(vin)
  Hybrid set/3(vno) -> Subsystem3/5(vno)
  I_st/1 -> Subsystem3/4(I_st)
  Subsystem3/1(v) -> vout/1
  Hybrid set/1(q) -> Subsystem3/1(q)
  Subsystem3/2(vnext) -> Event generator/1(v), Hybrid set/1(v)
  Hybrid set/2(vreset) -> Subsystem3/2(vreset)
  Hybrid set/4(reset) -> Subsystem3/3(reset)

== system heart_model/Heart Model/ATRIUM/Slow_a (31) ==
  stim : Inport
  I_st : Inport  Port=2
  vin : Inport  Port=3
  win : Inport  Port=4
  Data Type Conversion : DataTypeConversion  OutMin=[0]  OutMax=[1]  OutDataTypeStr=double  LockScale=on
  Data Type Conversion1 : DataTypeConversion  OutMin=[0]  OutMax=[1]  OutDataTypeStr=double  LockScale=on
  Data Type Conversion2 : DataTypeConversion  OutMin=[0]  OutMax=[1]  OutDataTypeStr=double  LockScale=on
  Event generator : Stateflow chart  TreatAsAtomicUnit=on
  Hybrid set : Stateflow chart  TreatAsAtomicUnit=on
  Mux : Mux  Inputs=5
  Subsystem3 : Subsystem
  vout : Outport
  wires:
  Data Type Conversion2/1 -> Mux/3
  Data Type Conversion1/1 -> Mux/2
  Event generator/3(event3) -> Data Type Conversion2/1
  Event generator/2(event2) -> Data Type Conversion1/1
  Data Type Conversion/1 -> Mux/1
  Event generator/1(event1) -> Data Type Conversion/1
  stim/1 -> Mux/5, Mux/4
  Mux/1 -> Hybrid set/Trigger
  win/1 -> Subsystem3/7(win)
  vin/1 -> Subsystem3/6(vin)
  Hybrid set/3(vno) -> Subsystem3/5(vno)
  I_st/1 -> Subsystem3/4(I_st)
  Subsystem3/1(v) -> vout/1
  Hybrid set/1(q) -> Subsystem3/1(q)
  Subsystem3/2(vnext) -> Event generator/1(v), Hybrid set/1(v)
  Hybrid set/2(vreset) -> Subsystem3/2(vreset)
  Hybrid set/4(reset) -> Subsystem3/3(reset)

== system heart_model/Heart Model/ATRIUM/Slow_b (30) ==
  stim : Inport
  I_st : Inport  Port=2
  vin : Inport  Port=3
  win : Inport  Port=4
  Data Type Conversion : DataTypeConversion  OutMin=[0]  OutMax=[1]  OutDataTypeStr=double  LockScale=on
  Data Type Conversion1 : DataTypeConversion  OutMin=[0]  OutMax=[1]  OutDataTypeStr=double  LockScale=on
  Data Type Conversion2 : DataTypeConversion  OutMin=[0]  OutMax=[1]  OutDataTypeStr=double  LockScale=on
  Event generator : Stateflow chart  TreatAsAtomicUnit=on
  Hybrid set : Stateflow chart  TreatAsAtomicUnit=on
  Mux : Mux  Inputs=5
  Subsystem3 : Subsystem
  vout : Outport
  wires:
  Data Type Conversion2/1 -> Mux/3
  Data Type Conversion1/1 -> Mux/2
  Event generator/3(event3) -> Data Type Conversion2/1
  Event generator/2(event2) -> Data Type Conversion1/1
  Data Type Conversion/1 -> Mux/1
  Event generator/1(event1) -> Data Type Conversion/1
  stim/1 -> Mux/5, Mux/4
  Mux/1 -> Hybrid set/Trigger
  win/1 -> Subsystem3/7(win)
  vin/1 -> Subsystem3/6(vin)
  Hybrid set/3(vno) -> Subsystem3/5(vno)
  I_st/1 -> Subsystem3/4(I_st)
  Subsystem3/1(v) -> vout/1
  Hybrid set/1(q) -> Subsystem3/1(q)
  Subsystem3/2(vnext) -> Event generator/1(v), Hybrid set/1(v)
  Hybrid set/2(vreset) -> Subsystem3/2(vreset)
  Hybrid set/4(reset) -> Subsystem3/3(reset)

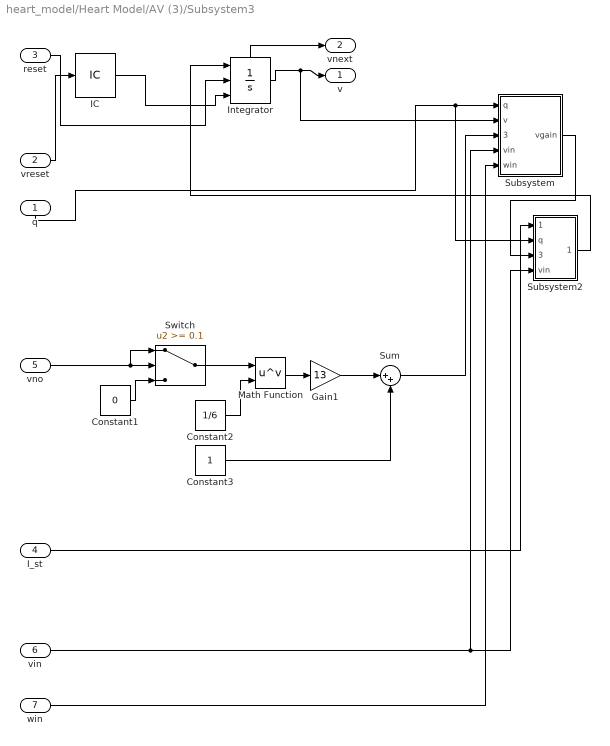
== system heart_model/Heart Model/AV (3)/Subsystem3 ==
  q : Inport
  vreset : Inport  Port=2
  reset : Inport  Port=3
  I_st : Inport  Port=4
  vno : Inport  Port=5
  vin : Inport  Port=6
  win : Inport  Port=7
  Constant1 : Constant  Value=0
  Constant2 : Constant  Value=1/6
  Constant3 : Constant
  Gain1 : Gain  Gain=13
  IC : InitialCondition  Value=0
  Integrator : Integrator  ExternalReset=either  InitialConditionSource=external  LimitOutput=on  UpperSaturationLimit=138  ShowStatePort=on
  Math Function : Math  Operator=pow  SaturateOnIntegerOverflow=on
  Subsystem : Subsystem
  Subsystem2 : Subsystem
  Sum : Sum  Inputs=|++
  Switch : Switch  Threshold=0.1
  v : Outport
  vnext : Outport  Port=2
  wires:
  win/1 -> Subsystem/5(win)
  vin/1 -> Subsystem/4(vin), Subsystem2/4(vin)
  Integrator/State -> vnext/1
  Constant1/1 -> Switch/3
  vno/1 -> Switch/1, Switch/2
  Sum/1 -> Subsystem/3(f(vno))
  Switch/1 -> Math Function/1
  Constant3/1 -> Sum/2
  Gain1/1 -> Sum/1
  Math Function/1 -> Gain1/1
  Constant2/1 -> Math Function/2
  I_st/1 -> Subsystem2/1(I_st)
  reset/1 -> Integrator/2
  vreset/1 -> IC/1
  Subsystem2/1(vint) -> Integrator/1
  Subsystem/1(vgain) -> Subsystem2/3(vgain)
  Integrator/1 -> Subsystem/2(v), v/1
  IC/1 -> Integrator/3
  q/1 -> Subsystem/1(q), Subsystem2/2(q)

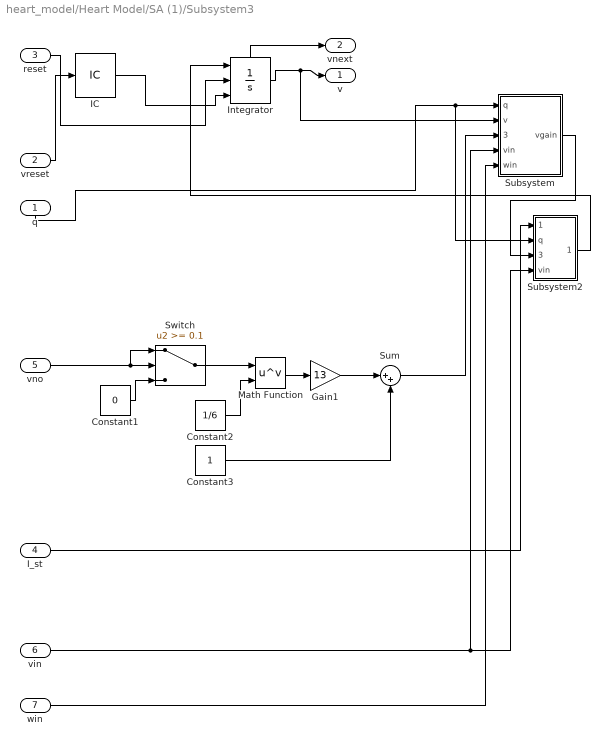
== system heart_model/Heart Model/SA (1)/Subsystem3 ==
  q : Inport
  vreset : Inport  Port=2
  reset : Inport  Port=3
  I_st : Inport  Port=4
  vno : Inport  Port=5
  vin : Inport  Port=6
  win : Inport  Port=7
  Constant1 : Constant  Value=0
  Constant2 : Constant  Value=1/6
  Constant3 : Constant
  Gain1 : Gain  Gain=13
  IC : InitialCondition  Value=0
  Integrator : Integrator  ExternalReset=either  InitialConditionSource=external  LimitOutput=on  UpperSaturationLimit=138  ShowStatePort=on
  Math Function : Math  Operator=pow  SaturateOnIntegerOverflow=on
  Subsystem : Subsystem
  Subsystem2 : Subsystem
  Sum : Sum  Inputs=|++
  Switch : Switch  Threshold=0.1
  v : Outport
  vnext : Outport  Port=2
  wires:
  win/1 -> Subsystem/5(win)
  vin/1 -> Subsystem/4(vin), Subsystem2/4(vin)
  Integrator/State -> vnext/1
  Constant1/1 -> Switch/3
  vno/1 -> Switch/1, Switch/2
  Sum/1 -> Subsystem/3(f(vno))
  Switch/1 -> Math Function/1
  Constant3/1 -> Sum/2
  Gain1/1 -> Sum/1
  Math Function/1 -> Gain1/1
  Constant2/1 -> Math Function/2
  I_st/1 -> Subsystem2/1(I_st)
  reset/1 -> Integrator/2
  vreset/1 -> IC/1
  Subsystem2/1(vint) -> Integrator/1
  Subsystem/1(vgain) -> Subsystem2/3(vgain)
  Integrator/1 -> Subsystem/2(v), v/1
  IC/1 -> Integrator/3
  q/1 -> Subsystem/1(q), Subsystem2/2(q)

== system heart_model/Heart Model/VENTRICLE/CS_LV (28) ==
  stim : Inport
  I_st : Inport  Port=2
  vin : Inport  Port=3
  win : Inport  Port=4
  Data Type Conversion : DataTypeConversion  OutMin=[0]  OutMax=[1]  OutDataTypeStr=double  LockScale=on
  Data Type Conversion1 : DataTypeConversion  OutMin=[0]  OutMax=[1]  OutDataTypeStr=double  LockScale=on
  Data Type Conversion2 : DataTypeConversion  OutMin=[0]  OutMax=[1]  OutDataTypeStr=double  LockScale=on
  Event generator : Stateflow chart  TreatAsAtomicUnit=on
  Hybrid set : Stateflow chart  TreatAsAtomicUnit=on
  Mux : Mux  Inputs=5
  Subsystem3 : Subsystem
  vout : Outport
  wires:
  Data Type Conversion2/1 -> Mux/3
  Data Type Conversion1/1 -> Mux/2
  Event generator/3(event3) -> Data Type Conversion2/1
  Event generator/2(event2) -> Data Type Conversion1/1
  Data Type Conversion/1 -> Mux/1
  Event generator/1(event1) -> Data Type Conversion/1
  stim/1 -> Mux/5, Mux/4
  Mux/1 -> Hybrid set/Trigger
  win/1 -> Subsystem3/7(win)
  vin/1 -> Subsystem3/6(vin)
  Hybrid set/3(vno) -> Subsystem3/5(vno)
  I_st/1 -> Subsystem3/4(I_st)
  Subsystem3/1(v) -> vout/1
  Hybrid set/1(q) -> Subsystem3/1(q)
  Subsystem3/2(vnext) -> Event generator/1(v), Hybrid set/1(v)
  Hybrid set/2(vreset) -> Subsystem3/2(vreset)
  Hybrid set/4(reset) -> Subsystem3/3(reset)

== system heart_model/Heart Model/VENTRICLE/His_d (7) ==
  stim : Inport
  I_st : Inport  Port=2
  vin : Inport  Port=3
  win : Inport  Port=4
  Data Type Conversion : DataTypeConversion  OutMin=[0]  OutMax=[1]  OutDataTypeStr=double  LockScale=on
  Data Type Conversion1 : DataTypeConversion  OutMin=[0]  OutMax=[1]  OutDataTypeStr=double  LockScale=on
  Data Type Conversion2 : DataTypeConversion  OutMin=[0]  OutMax=[1]  OutDataTypeStr=double  LockScale=on
  Event generator : Stateflow chart  TreatAsAtomicUnit=on
  Hybrid set : Stateflow chart  TreatAsAtomicUnit=on
  Mux : Mux  Inputs=5
  Subsystem3 : Subsystem
  vout : Outport
  wires:
  Data Type Conversion2/1 -> Mux/3
  Data Type Conversion1/1 -> Mux/2
  Event generator/3(event3) -> Data Type Conversion2/1
  Event generator/2(event2) -> Data Type Conversion1/1
  Data Type Conversion/1 -> Mux/1
  Event generator/1(event1) -> Data Type Conversion/1
  stim/1 -> Mux/5, Mux/4
  Mux/1 -> Hybrid set/Trigger
  win/1 -> Subsystem3/7(win)
  vin/1 -> Subsystem3/6(vin)
  Hybrid set/3(vno) -> Subsystem3/5(vno)
  I_st/1 -> Subsystem3/4(I_st)
  Subsystem3/1(v) -> vout/1
  Hybrid set/1(q) -> Subsystem3/1(q)
  Subsystem3/2(vnext) -> Event generator/1(v), Hybrid set/1(v)
  Hybrid set/2(vreset) -> Subsystem3/2(vreset)
  Hybrid set/4(reset) -> Subsystem3/3(reset)

== system heart_model/Heart Model/VENTRICLE/His_m (6) ==
  stim : Inport
  I_st : Inport  Port=2
  vin : Inport  Port=3
  win : Inport  Port=4
  Data Type Conversion : DataTypeConversion  OutMin=[0]  OutMax=[1]  OutDataTypeStr=double  LockScale=on
  Data Type Conversion1 : DataTypeConversion  OutMin=[0]  OutMax=[1]  OutDataTypeStr=double  LockScale=on
  Data Type Conversion2 : DataTypeConversion  OutMin=[0]  OutMax=[1]  OutDataTypeStr=double  LockScale=on
  Event generator : Stateflow chart  TreatAsAtomicUnit=on
  Hybrid set : Stateflow chart  TreatAsAtomicUnit=on
  Mux : Mux  Inputs=5
  Subsystem3 : Subsystem
  vout : Outport
  wires:
  Data Type Conversion2/1 -> Mux/3
  Data Type Conversion1/1 -> Mux/2
  Event generator/3(event3) -> Data Type Conversion2/1
  Event generator/2(event2) -> Data Type Conversion1/1
  Data Type Conversion/1 -> Mux/1
  Event generator/1(event1) -> Data Type Conversion/1
  stim/1 -> Mux/5, Mux/4
  Mux/1 -> Hybrid set/Trigger
  win/1 -> Subsystem3/7(win)
  vin/1 -> Subsystem3/6(vin)
  Hybrid set/3(vno) -> Subsystem3/5(vno)
  I_st/1 -> Subsystem3/4(I_st)
  Subsystem3/1(v) -> vout/1
  Hybrid set/1(q) -> Subsystem3/1(q)
  Subsystem3/2(vnext) -> Event generator/1(v), Hybrid set/1(v)
  Hybrid set/2(vreset) -> Subsystem3/2(vreset)
  Hybrid set/4(reset) -> Subsystem3/3(reset)

== system heart_model/Heart Model/VENTRICLE/His_p (5) ==
  stim : Inport
  I_st : Inport  Port=2
  vin : Inport  Port=3
  win : Inport  Port=4
  Data Type Conversion : DataTypeConversion  OutMin=[0]  OutMax=[1]  OutDataTypeStr=double  LockScale=on
  Data Type Conversion1 : DataTypeConversion  OutMin=[0]  OutMax=[1]  OutDataTypeStr=double  LockScale=on
  Data Type Conversion2 : DataTypeConversion  OutMin=[0]  OutMax=[1]  OutDataTypeStr=double  LockScale=on
  Event generator : Stateflow chart  TreatAsAtomicUnit=on
  Hybrid set : Stateflow chart  TreatAsAtomicUnit=on
  Mux : Mux  Inputs=5
  Subsystem3 : Subsystem
  vout : Outport
  wires:
  Data Type Conversion2/1 -> Mux/3
  Data Type Conversion1/1 -> Mux/2
  Event generator/3(event3) -> Data Type Conversion2/1
  Event generator/2(event2) -> Data Type Conversion1/1
  Data Type Conversion/1 -> Mux/1
  Event generator/1(event1) -> Data Type Conversion/1
  stim/1 -> Mux/5, Mux/4
  Mux/1 -> Hybrid set/Trigger
  win/1 -> Subsystem3/7(win)
  vin/1 -> Subsystem3/6(vin)
  Hybrid set/3(vno) -> Subsystem3/5(vno)
  I_st/1 -> Subsystem3/4(I_st)
  Subsystem3/1(v) -> vout/1
  Hybrid set/1(q) -> Subsystem3/1(q)
  Subsystem3/2(vnext) -> Event generator/1(v), Hybrid set/1(v)
  Hybrid set/2(vreset) -> Subsystem3/2(vreset)
  Hybrid set/4(reset) -> Subsystem3/3(reset)

== system heart_model/Heart Model/VENTRICLE/LBB (14) ==
  stim : Inport
  I_st : Inport  Port=2
  vin : Inport  Port=3
  win : Inport  Port=4
  Data Type Conversion : DataTypeConversion  OutMin=[0]  OutMax=[1]  OutDataTypeStr=double  LockScale=on
  Data Type Conversion1 : DataTypeConversion  OutMin=[0]  OutMax=[1]  OutDataTypeStr=double  LockScale=on
  Data Type Conversion2 : DataTypeConversion  OutMin=[0]  OutMax=[1]  OutDataTypeStr=double  LockScale=on
  Event generator : Stateflow chart  TreatAsAtomicUnit=on
  Hybrid set : Stateflow chart  TreatAsAtomicUnit=on
  Mux : Mux  Inputs=5
  Subsystem3 : Subsystem
  vout : Outport
  wires:
  Data Type Conversion2/1 -> Mux/3
  Data Type Conversion1/1 -> Mux/2
  Event generator/3(event3) -> Data Type Conversion2/1
  Event generator/2(event2) -> Data Type Conversion1/1
  Data Type Conversion/1 -> Mux/1
  Event generator/1(event1) -> Data Type Conversion/1
  stim/1 -> Mux/5, Mux/4
  Mux/1 -> Hybrid set/Trigger
  win/1 -> Subsystem3/7(win)
  vin/1 -> Subsystem3/6(vin)
  Hybrid set/3(vno) -> Subsystem3/5(vno)
  I_st/1 -> Subsystem3/4(I_st)
  Subsystem3/1(v) -> vout/1
  Hybrid set/1(q) -> Subsystem3/1(q)
  Subsystem3/2(vnext) -> Event generator/1(v), Hybrid set/1(v)
  Hybrid set/2(vreset) -> Subsystem3/2(vreset)
  Hybrid set/4(reset) -> Subsystem3/3(reset)

== system heart_model/Heart Model/VENTRICLE/LBB_m (13) ==
  stim : Inport
  I_st : Inport  Port=2
  vin : Inport  Port=3
  win : Inport  Port=4
  Data Type Conversion : DataTypeConversion  OutMin=[0]  OutMax=[1]  OutDataTypeStr=double  LockScale=on
  Data Type Conversion1 : DataTypeConversion  OutMin=[0]  OutMax=[1]  OutDataTypeStr=double  LockScale=on
  Data Type Conversion2 : DataTypeConversion  OutMin=[0]  OutMax=[1]  OutDataTypeStr=double  LockScale=on
  Event generator : Stateflow chart  TreatAsAtomicUnit=on
  Hybrid set : Stateflow chart  TreatAsAtomicUnit=on
  Mux : Mux  Inputs=5
  Subsystem3 : Subsystem
  vout : Outport
  wires:
  Data Type Conversion2/1 -> Mux/3
  Data Type Conversion1/1 -> Mux/2
  Event generator/3(event3) -> Data Type Conversion2/1
  Event generator/2(event2) -> Data Type Conversion1/1
  Data Type Conversion/1 -> Mux/1
  Event generator/1(event1) -> Data Type Conversion/1
  stim/1 -> Mux/5, Mux/4
  Mux/1 -> Hybrid set/Trigger
  win/1 -> Subsystem3/7(win)
  vin/1 -> Subsystem3/6(vin)
  Hybrid set/3(vno) -> Subsystem3/5(vno)
  I_st/1 -> Subsystem3/4(I_st)
  Subsystem3/1(v) -> vout/1
  Hybrid set/1(q) -> Subsystem3/1(q)
  Subsystem3/2(vnext) -> Event generator/1(v), Hybrid set/1(v)
  Hybrid set/2(vreset) -> Subsystem3/2(vreset)
  Hybrid set/4(reset) -> Subsystem3/3(reset)
